simulink model "hw55"  (R2020b)
settings: Solver=VariableStepAuto  StartTime=0.0  StopTime=10.0  RelTol=1e-3
libraries: simulink x1
settings Model: Creator=Lee  LastModifiedBy=Lee

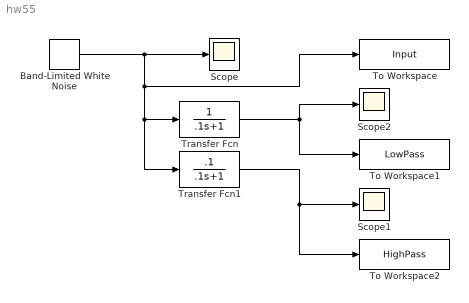
== system hw55 ==
  Band-Limited White Noise : simulink/Sources/Band-Limited White Noise  Cov=[0.1]  Ts=0.1  seed=[23341]
  Scope : Scope
  Scope1 : Scope
  Scope2 : Scope
  To Workspace : ToWorkspace  VariableName=Input  SaveFormat=Timeseries  SampleTime=-1
  To Workspace1 : ToWorkspace  VariableName=LowPass  SaveFormat=Timeseries  SampleTime=-1
  To Workspace2 : ToWorkspace  VariableName=HighPass  SaveFormat=Timeseries  SampleTime=-1
  Transfer Fcn : TransferFcn  Denominator=[.1 1]
  Transfer Fcn1 : TransferFcn  Numerator=[.1]  Denominator=[.1 1]
  wires:
  Band-Limited White Noise/1 -> To Workspace/1, Transfer Fcn/1, Transfer Fcn1/1, Scope/1
  Transfer Fcn1/1 -> To Workspace2/1, Scope1/1
  Transfer Fcn/1 -> Scope2/1, To Workspace1/1
